simulink model "SistemaCompleto_PMSM"  (R2023b)
settings: Solver=VariableStepAuto  StartTime=0.0  StopTime=2  RelTol=1e-3
PostLoadFcn:
  | parametros_sistema_completo
  | run("parametros_sistema_completo.mlx")
values from neighbouring files (symbols this model uses):
  a_cu = 3.9e-3    (= 0.0039)    [parametros_sistema_completo.m]    (also in workspace_params.mat)
  A_i = [0,  1,                          0 ... (first row only)    [analisis_estabilidad_LA.m]
  b_eq = params.b_total    [calcular_matriz_AO.m]    (also in calculo_incertidumbre_y_control.m = b_m + b_l/(r^2); parametros_sistema_completo.m = 2.19444444444e-05; workspace_params.mat = 2.19444444444e-05)
  C_ts = C_ts * (1 + tol_pct)    [calculo_incertidumbre_y_control.m]    (also in parametros_sistema_completo.m = 0.818; workspace_params.mat = 0.818)
  g = 9.80665    [parametros_sistema_completo.m]    (also in workspace_params.mat)
  J_eq = params.J_total    [calcular_matriz_AO.m]    (also in calculo_incertidumbre_y_control.m = J_m + J_l/r^2; parametros_sistema_completo.m = 1.97847222222e-05; workspace_params.mat = 3.28055555556e-05)
  k_l = m*l_cm + m_l*l_l    [calculo_incertidumbre_y_control.m]    (also in parametros_sistema_completo.m = 0.25; workspace_params.mat = 0.625)
  L_d = L_d    * (1 - tol_pct)    [calculo_incertidumbre_y_control.m]    (also in parametros_sistema_completo.m = 0.0066; workspace_params.mat = 0.0066)
  L_ls = L_ls   * (1 - tol_pct)    [calculo_incertidumbre_y_control.m]    (also in parametros_sistema_completo.m = 0.0008; workspace_params.mat = 0.0008)
  L_q = L_q    * (1 - tol_pct)    [calculo_incertidumbre_y_control.m]    (also in parametros_sistema_completo.m = 0.0058; workspace_params.mat = 0.0058)
  lambda_r = lambda_r * (1 + tol_pct)    [calculo_incertidumbre_y_control.m]    (also in parametros_sistema_completo.m = 0.016; workspace_params.mat = 0.016)
  P_p = 3    [parametros_sistema_completo.m]    (also in workspace_params.mat)
  params = struct()    [evaluar_migracion_Ids.m]    (also in parametros_sistema_completo.m; workspace_params.mat = )
  r = params.r_red    [calcular_matriz_AO.m]    (also in parametros_sistema_completo.m = 120; workspace_params.mat = 120)
  R_s_sim = R_sREF * (1 + a_cu * (T_s_sim - T_sREF))    [configurar_temperatura_516.m]
  R_sREF = R_sREF * (1 - tol_pct)    [calculo_incertidumbre_y_control.m]    (also in parametros_sistema_completo.m = 1.02; workspace_params.mat = 1.02)
  R_ts_amb = R_ts_amb * (1 - tol_pct)    [calculo_incertidumbre_y_control.m]    (also in parametros_sistema_completo.m = 146.7; workspace_params.mat = 146.7)
  T_amb = 20    [parametros_sistema_completo.m]    (also in workspace_params.mat)
  T_s = x(6)    [modulador_torque_521.m]    (also in simulacion_dinamica_516.m)
  T_sREF = 20    [parametros_sistema_completo.m]    (also in workspace_params.mat)
undefined symbols (not defined in the file or in its folder): A_T, A_theta, A_v, b_a, B_i, B_T, B_theta, B_v, C_i, C_T, C_theta, C_v, consigna_posicion, D_i, D_T, D_theta, D_v, i_ds_inicial, Is_pico, Is_rms_max, Is_rms_nom, K_e_i_m_int, K_e_tita_m, K_e_tita_m_int, K_e_w_m, K_e_w_m_int, K_p0, K_pd, K_pq, K_sa, K_sia, pos_inicial, t_rampa_acel, t_rampa_vel, V_sl_max, x0_ias, x0_ibs, x0_ics, x0_T, x0_theta
libraries: simulink_extras x8, SignalEditorBlockLib x6, eeStairGenerator x4, simulink x1
(part 7 of 7)

== matlab function SistemaCompleto_PMSM/Modelo Global NL perfil trapezoidal aceleracion y codificado/Controlador/MATLAB Function ==
  settings: updateMethod=DISCRETE  sampleTime=1e-4
  data: t input; theta_ref output; omega_ref output; consigna_posicion parameter size=[4 2]; t_rampa_vel parameter; t_rampa_acel parameter; accel_ref output
function [theta_ref,omega_ref,accel_ref]= GeneradorTrayectoria(t,consigna_posicion, t_rampa_vel, t_rampa_acel)
persistent inicializado
persistent dt_vec dq_vec
persistent h1_vec h2_vec
persistent tr1_vec tr2_vec
persistent t_nodos q_nodos N

if isempty(inicializado)
    N = 0;
    for i = 1:size(consigna_posicion,1)
        if ~isnan(consigna_posicion(i,1)) && ~isnan(consigna_posicion(i,2))
            N = N + 1;
        else
            break;
        end
    end

    if N < 2
        error('Debe haber al menos 2 puntos válidos en Matriz_Consigna');
    end
    t_nodos = consigna_posicion(1:N,1);
    q_nodos = consigna_posicion(1:N,2);
    n_tramos = N-1;
    dt_vec = zeros(n_tramos,1);
    dq_vec = zeros(n_tramos,1);
    h1_vec = zeros(n_tramos,1);
    h2_vec = zeros(n_tramos,1);
    tr1_vec = zeros(n_tramos,1);
    tr2_vec = zeros(n_tramos,1);
    for k = 1:n_tramos
        dt_vec(k) = t_nodos(k+1)-t_nodos(k);
        dq_vec(k) = q_nodos(k+1)-q_nodos(k);

        tr1_vec(k)=t_rampa_vel;
        tr2_vec(k)=t_rampa_acel;

        if tr1_vec(k) <= 0
            error('t_rampa_vel debe ser > 0 en el tramo %d.',k);
        end

        if tr2_vec(k) <= 0 || tr2_vec(k) >= tr1_vec(k)
            error('Debe cumplirse 0 < t_rampa_acel < t_rampa_vel en el tramo %d.',k);
        end

        if dt_vec(k) < 2*tr1_vec(k)
            error('Debe cumplirse dt >= 2*t_rampa_vel en el tramo %d.',k);
        end
        %Altura velocidad
        h1_vec(k) = abs(dq_vec(k))/(dt_vec(k)-tr1_vec(k));
        h2_vec(k) = h1_vec(k)/(tr1_vec(k)-tr2_vec(k));
    end
    inicializado=true;
end

if t <= t_nodos(1)
    theta_ref = q_nodos(1);
    omega_ref = 0;
    accel_ref = 0;
    return;
end

if t>= t_nodos(end)
    theta_ref = q_nodos(end);
    omega_ref = 0;
    accel_ref = 0;
    return;
end

tramo_actual = 1;
for k = 1:(N-1)
    if t >= t_nodos(k) && t < t_nodos(k+1)
        tramo_actual = k;
        break;
    end
end
tau = t - t_nodos(tramo_actual);

q0  = q_nodos(tramo_actual);
dt  = dt_vec(tramo_actual);
dq  = dq_vec(tramo_actual);
h1  = h1_vec(tramo_actual);
h2  = h2_vec(tramo_actual);
tr1 = tr1_vec(tramo_actual);
tr2 = tr2_vec(tramo_actual);
sgn = sign(dq);
dq_abs = abs(dq);
if dq_abs < 1e-12
    theta_ref = q0;
    omega_ref = 0;
    accel_ref = 0;
    return;
end

% if tau < tr1
%     % Aceleración
%     omega_ref = h1 * (tau / tr1);
%     theta_ref = q0 + 0.5 * (h1/tr1) * tau^2;
% elseif tau < (dt - tr1)
%     % Velocidad constante
%     omega_ref = h1;
%     theta_ref = q0 ...
%         + 0.5*h1*tr1 ...
%         + h1*(tau - tr1);
%
% elseif tau <= dt
%     % Desaceleración
%     td = tau - (dt - tr1);
%     omega_ref = h1 * (1 - td/tr1);
%     theta_ref = q_nodos(tramo_actual+1) ...
%         - 0.5 * (h1/tr1) * (dt - tau)^2;
% else
%     theta_ref = q_nodos(tramo_actual+1);
%     omega_ref = 0;
% end

[theta_ref, omega_ref, accel_ref] = perfil_7_subtramos( ...
    tau, q0, q_nodos(tramo_actual+1), dt, h1, h2, tr1, tr2, sgn);
end

function [theta_ref, omega_ref, accel_ref] = perfil_7_subtramos(tau, q0, qf, dt, h1, h2, tr1, tr2, sgn)

    d_acc = 0.5*h1*tr1;

    if tau <= 0
        theta_ref = q0;
        omega_ref = 0;
        accel_ref = 0;

    elseif tau < tr1
        [s_local, w_local, a_local] = perfil_arranque_local(tau, h2, tr1, tr2);
        theta_ref = q0 + sgn*s_local;
        omega_ref = sgn*w_local;
        accel_ref = sgn*a_local;

    elseif tau < (dt - tr1)
        u = tau - tr1;
        theta_ref = q0 + sgn*(d_acc + h1*u);
        omega_ref = sgn*h1;
        accel_ref = 0;

    elseif tau <= dt
        rho = dt - tau;
        [s_local, w_local, a_local] = perfil_arranque_local(rho, h2, tr1, tr2);
        theta_ref = qf - sgn*s_local;
        omega_ref = sgn*w_local;
        accel_ref = -sgn*a_local;

    else
        theta_ref = qf;
        omega_ref = 0;
        accel_ref = 0;
    end
end
function [s_local, w_local, a_local] = perfil_arranque_local(tloc, h2, tr1, tr2)

    t1 = tr2;
    t2 = tr1 - tr2;

    if tloc <= 0
        s_local = 0;
        w_local = 0;
        a_local = 0;

    elseif tloc < t1
        % Subtramo 1: aceleración sube linealmente
        a_local = (h2/tr2)*tloc;
        w_local = (h2/(2*tr2))*tloc^2;
        s_local = (h2/(6*tr2))*tloc^3;

    elseif tloc < t2
        % Subtramo 2: aceleración constante = h2
        u = tloc - tr2;

        w1 = h2*tr2/2;
        s1 = h2*tr2^2/6;

        a_local = h2;
        w_local = w1 + h2*u;
        s_local = s1 + w1*u + 0.5*h2*u^2;

    elseif tloc <= tr1
        % Subtramo 3: aceleración baja linealmente hasta 0
        u = tloc - (tr1 - tr2);

        w2 = h2*tr2/2 + h2*(tr1 - 2*tr2);
        s2 = h2*tr2^2/6 ...
           + (h2*tr2/2)*(tr1 - 2*tr2) ...
           + 0.5*h2*(tr1 - 2*tr2)^2;

        a_local = h2 - (h2/tr2)*u;
        w_local = w2 + h2*u - (h2/(2*tr2))*u^2;
        s_local = s2 + w2*u + 0.5*h2*u^2 - (h2/(6*tr2))*u^3;

    else
        a_local = 0;
        w_local = h2*(tr1 - tr2);   % = h1
        s_local = 0.5*w_local*tr1;
    end
end

== matlab function SistemaCompleto_PMSM/Modelo Global NL perfil trapezoidal aceleracion y codificado/Controlador/Controlador PID de Posicion/MATLAB Function1 ==
  data: e_wm input; Tm output; params input
function Tm = controladorPosicion(e_wm,params)
% Calcula la orden de par Tm** en función del error de velocidad e_wm[k]
% usando integradores discretos tipo Tustin.
%
% Variables que se leen del workspace:
%   Ts   – periodo de muestreo
%   b_a  – ganancia del término proporcional (error de velocidad)
%   K_sa – ganancia del primer integrador (error de posición)
%   K_sia– ganancia del segundo integrador

    Ts   = params.Ts;
    b_a  = params.b_a;
    K_sa = params.K_sa;
    K_sia= params.K_sia;
    % Variables persistentes para almacenar estados entre llamadas
    persistent e_theta_prev e_theta_int_prev e_prev
    if isempty(e_theta_prev)
        e_theta_prev    = 0;   % integral del error de velocidad en k‑1
        e_theta_int_prev= 0;   % doble integral en k‑1
        e_prev          = 0;   % error de velocidad en k‑1
    end

    % Primer integrador (Tustin): integra e_wm
    e_theta = e_theta_prev + (Ts/2)*(e_wm + e_prev);

    % Segundo integrador (Tustin): integra e_theta
    e_theta_int = e_theta_int_prev + (Ts/2)*(e_theta + e_theta_prev);

    % Cálculo del par de referencia
    Tm = b_a*e_wm + K_sa*e_theta + K_sia*e_theta_int;

    % Actualizar estados para la próxima llamada
    e_prev           = e_wm;
    e_theta_prev     = e_theta;
    e_theta_int_prev = e_theta_int;
end
